simulink model "TraditionalStarterGenerator"  (R2024b)
settings: Solver=VariableStepAuto  StartTime=0.0  StopTime=20  MaxStep=1  RelTol=1e-3  EnableMultiTasking=on
undefined symbols (not defined in the file or in its folder): DiscIntNeverNeededParam
libraries: fl_lib x47, fl_ps_legacy_lib x26, ee_lib x25, nesl_utility x17, sdl_lib x1, SignalEditorBlockLib x1
(part 2 of 2)

== system TraditionalStarterGenerator/loads/Low Beam ==
  Fuse Right : ee_lib/Switches & Breakers/Fuse  prm=1  I_rated=15 A  melt_margin=1  T_fuse=0.5 s  I2t=1 s*A^2  I_vec=[1.9, 2.0, 2.5, 30.0] A  t_vec=[10000.0, 1.0, 0.3, 0.001] s  R_closed=0.01 Ohm  G_open=1e-8 1/Ohm  exposemeasurement=ee.enum.exposemeasurement.hidden
      settings: AttributesFormatString=%<I_rated> %<I_rated_unit>  InternalSimscapePortConfiguration="{\"Bottom\":[],\"Left\":[{\"id\":\"p\",\"label\":\"\",\"type\":\"foundation.electrical.electrical\"}],\"Right\":[{\"id\":\"n\",\"label\":\"\",\"type\":\"foundation.electrical.electrical\"}],\"Top\":[]}"
  Lamp : ee_lib/Passive/Incandescent Lamp  R_param=2  R0=0.15 Ohm  R1=1 Ohm  i0=5*25/12 A  i1=25/12 A  Vrated=12 V  alpha=0.004 1/K  tc=25 ms  initial_state=simscape.enum.onoff.off  t_fault=inf s
      settings: InternalSimscapePortConfiguration="{\"Bottom\":[],\"Left\":[{\"id\":\"p\",\"label\":\"+\",\"type\":\"foundation.electrical.electrical\"}],\"Right\":[{\"id\":\"n\",\"label\":\"-\",\"type\":\"foundation.electrical.electrical\"}],\"Top\":[]}"
  SPST Switch : ee_lib/Switches & Breakers/SPST Switch  R_closed=0.01 Ohm  G_open=1e-6 S  Threshold=0.5 V  Width=0 V  model_dynamics=0  t_on=1e-3 s  t_off=1e-3 s  initial_vT=0 V
      settings: InternalSimscapePortConfiguration="{\"Bottom\":[],\"Left\":[{\"id\":\"vT\",\"label\":\"vT\",\"type\":\"input\"},{\"id\":\"p\",\"label\":\"\",\"type\":\"foundation.electrical.electrical\"}],\"Right\":[{\"id\":\"n\",\"label\":\"\",\"type\":\"foundation.electrical.electrical\"}],\"Top\":[]}"
  Switch : PMIOPort  Side=Left
  - : PMIOPort  Port=2  Side=Right
  + : PMIOPort  Port=3  Side=Left
  connections:
  Fuse Right/RConn1 -- SPST Switch/LConn2
  SPST Switch/LConn1 -- Switch/RConn1
  SPST Switch/RConn1 -- Lamp/LConn1
  +/RConn1 -- Fuse Right/LConn1
  Lamp/RConn1 -- -/RConn1

== system TraditionalStarterGenerator/loads/Subsystem2 ==
  Simulink-PS Converter : nesl_utility/Simulink-PS Converter  PhysicalDomain=network_engine_domain  SubClassName=ps_input  LeftPortType=input  RightPortType=output  PseudoPeriodic=off  Frequencies=[]  NoiseDistribution=none  NoiseParameters=[]  Unit=1  AffineConversion=off  FilteringAndDerivatives=zero  SimscapeFilterOrder=1  InputFilterTimeConstant=0.001  UdotUserProvided=1
  ind_L : PMIOPort  Side=Right
  wires:
  [ind_L] -> Simulink-PS Converter/1
  connections:
  Simulink-PS Converter/RConn1 -- ind_L/RConn1

== system TraditionalStarterGenerator/loads/Subsystem3 ==
  Simulink-PS Converter : nesl_utility/Simulink-PS Converter  PhysicalDomain=network_engine_domain  SubClassName=ps_input  LeftPortType=input  RightPortType=output  PseudoPeriodic=off  Frequencies=[]  NoiseDistribution=none  NoiseParameters=[]  Unit=1  AffineConversion=off  FilteringAndDerivatives=zero  SimscapeFilterOrder=1  InputFilterTimeConstant=0.001  UdotUserProvided=1
  ind_R : PMIOPort  Side=Right
  wires:
  [ind_R] -> Simulink-PS Converter/1
  connections:
  Simulink-PS Converter/RConn1 -- ind_R/RConn1

== system TraditionalStarterGenerator/loads/Subsystem4 ==
  Simulink-PS Converter : nesl_utility/Simulink-PS Converter  PhysicalDomain=network_engine_domain  SubClassName=ps_input  LeftPortType=input  RightPortType=output  PseudoPeriodic=off  Frequencies=[]  NoiseDistribution=none  NoiseParameters=[]  Unit=1  AffineConversion=off  FilteringAndDerivatives=zero  SimscapeFilterOrder=1  InputFilterTimeConstant=0.001  UdotUserProvided=1
  lights : PMIOPort  Side=Right
  wires:
  [lights] -> Simulink-PS Converter/1
  connections:
  Simulink-PS Converter/RConn1 -- lights/RConn1

== system TraditionalStarterGenerator/loads/Subsystem5 ==
  Simulink-PS Converter : nesl_utility/Simulink-PS Converter  PhysicalDomain=network_engine_domain  SubClassName=ps_input  LeftPortType=input  RightPortType=output  PseudoPeriodic=off  Frequencies=[]  NoiseDistribution=none  NoiseParameters=[]  Unit=1  AffineConversion=off  FilteringAndDerivatives=zero  SimscapeFilterOrder=1  InputFilterTimeConstant=0.001  UdotUserProvided=1
  lights : PMIOPort  Side=Right
  wires:
  [lights] -> Simulink-PS Converter/1
  connections:
  Simulink-PS Converter/RConn1 -- lights/RConn1

== system TraditionalStarterGenerator/loads/Subsystem6 ==
  Simulink-PS Converter : nesl_utility/Simulink-PS Converter  PhysicalDomain=network_engine_domain  SubClassName=ps_input  LeftPortType=input  RightPortType=output  PseudoPeriodic=off  Frequencies=[]  NoiseDistribution=none  NoiseParameters=[]  Unit=1  AffineConversion=off  FilteringAndDerivatives=zero  SimscapeFilterOrder=1  InputFilterTimeConstant=0.001  UdotUserProvided=1
  brake : PMIOPort  Side=Right
  wires:
  [brake] -> Simulink-PS Converter/1
  connections:
  Simulink-PS Converter/RConn1 -- brake/RConn1

== system TraditionalStarterGenerator/loads/Subsystem7 ==
  Simulink-PS Converter : nesl_utility/Simulink-PS Converter  PhysicalDomain=network_engine_domain  SubClassName=ps_input  LeftPortType=input  RightPortType=output  PseudoPeriodic=off  Frequencies=[]  NoiseDistribution=none  NoiseParameters=[]  Unit=1  AffineConversion=off  FilteringAndDerivatives=zero  SimscapeFilterOrder=1  InputFilterTimeConstant=0.001  UdotUserProvided=1
  beam : PMIOPort  Side=Right
  wires:
  [beam] -> Simulink-PS Converter/1
  connections:
  Simulink-PS Converter/RConn1 -- beam/RConn1

== system TraditionalStarterGenerator/loads/Tail Light ==
  Fuse : ee_lib/Switches & Breakers/Fuse  prm=1  I_rated=5 A  melt_margin=1  T_fuse=0.5 s  I2t=1 s*A^2  I_vec=[1.9, 2.0, 2.5, 30.0] A  t_vec=[10000.0, 1.0, 0.3, 0.001] s  R_closed=0.01 Ohm  G_open=1e-8 1/Ohm  exposemeasurement=ee.enum.exposemeasurement.hidden
      settings: AttributesFormatString=%<I_rated> %<I_rated_unit>  InternalSimscapePortConfiguration="{\"Bottom\":[],\"Left\":[{\"id\":\"p\",\"label\":\"\",\"type\":\"foundation.electrical.electrical\"}],\"Right\":[{\"id\":\"n\",\"label\":\"\",\"type\":\"foundation.electrical.electrical\"}],\"Top\":[]}"
  Lamp : ee_lib/Passive/Incandescent Lamp  R_param=2  R0=0.15 Ohm  R1=1 Ohm  i0=5*5/12 A  i1=5/12 A  Vrated=12 V  alpha=0.004 1/K  tc=25 ms  initial_state=simscape.enum.onoff.off  t_fault=inf s
      settings: InternalSimscapePortConfiguration="{\"Bottom\":[],\"Left\":[{\"id\":\"p\",\"label\":\"+\",\"type\":\"foundation.electrical.electrical\"}],\"Right\":[{\"id\":\"n\",\"label\":\"-\",\"type\":\"foundation.electrical.electrical\"}],\"Top\":[]}"
  Switch SPST : ee_lib/Switches & Breakers/SPST Switch  R_closed=1 Ohm  G_open=1e-6 S  Threshold=0.5 V  Width=0 V  model_dynamics=0  t_on=0.001 s  t_off=0.001 s  initial_vT=0 V
      settings: InternalSimscapePortConfiguration="{\"Bottom\":[],\"Left\":[{\"id\":\"vT\",\"label\":\"vT\",\"type\":\"input\"},{\"id\":\"p\",\"label\":\"\",\"type\":\"foundation.electrical.electrical\"}],\"Right\":[{\"id\":\"n\",\"label\":\"\",\"type\":\"foundation.electrical.electrical\"}],\"Top\":[]}"
  Switch : PMIOPort  Side=Left
  + : PMIOPort  Port=2  Side=Left
  - : PMIOPort  Port=3  Side=Right
  connections:
  +/RConn1 -- Fuse/LConn1
  Lamp/RConn1 -- -/RConn1
  Switch/RConn1 -- Switch SPST/LConn1
  Fuse/RConn1 -- Switch SPST/LConn2
  Switch SPST/RConn1 -- Lamp/LConn1

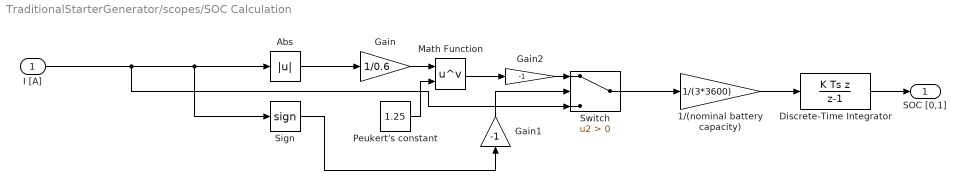
== system TraditionalStarterGenerator/scopes/SOC Calculation ==
  I [A] : Inport
  1/(nominal battery capacity) : Gain  Gain=1/(3*3600)
  Abs : Abs  SaturateOnIntegerOverflow=off
  Discrete-Time Integrator : DiscreteIntegrator  IntegratorMethod=Integration: Backward Euler  InitialCondition=0.5  SampleTime=0.0001  LimitOutput=on  UpperSaturationLimit=1  LowerSaturationLimit=0  ICPrevOutput=DiscIntNeverNeededParam  ICPrevScaledInput=DiscIntNeverNeededParam
  Gain : Gain  Gain=1/0.6
  Gain1 : Gain  Gain=-1
  Gain2 : Gain  Gain=-1
  Math Function : Math  Operator=pow
  Peukert's constant : Constant  Value=1.25  SampleTime=-1
  Sign : Signum
  Switch : Switch  Criteria=u2 > Threshold  SaturateOnIntegerOverflow=off  InputSameDT=off
  SOC [0,1] : Outport  VectorParamsAs1DForOutWhenUnconnected=off
  wires:
  Gain2/1 -> Switch/1
  Abs/1 -> Gain/1
  Discrete-Time Integrator/1 -> SOC [0,1]/1
  Sign/1 -> Gain1/1
  Math Function/1 -> Gain2/1
  I [A]/1 -> Sign/1, Abs/1, Switch/3
  Peukert's constant/1 -> Math Function/2
  Gain/1 -> Math Function/1
  Gain1/1 -> Switch/2
  Switch/1 -> 1/(nominal battery capacity)/1
  1/(nominal battery capacity)/1 -> Discrete-Time Integrator/1

== system TraditionalStarterGenerator/Alternator/Back EMF and Torque/Current Voltage Interface ==
  Controlled Voltage Source : fl_lib/Electrical/Electrical Sources/Controlled Voltage Source
  Current Sensor : fl_lib/Electrical/Electrical Sensors/Current Sensor
  v : PMIOPort  Side=Left
  i : PMIOPort  Port=2  Side=Right
  + : PMIOPort  Port=3  Side=Left
  - : PMIOPort  Port=4  Side=Right
  connections:
  Current Sensor/RConn1 -- i/RConn1
  Controlled Voltage Source/RConn1 -- v/RConn1
  Current Sensor/RConn2 -- Controlled Voltage Source/RConn2
  -/RConn1 -- Current Sensor/LConn1
  +/RConn1 -- Controlled Voltage Source/LConn1

== system TraditionalStarterGenerator/Alternator/Back EMF and Torque/Torque Motion Interface ==
  Motion Sensor : fl_lib/Mechanical/Mechanical Sensors/Ideal Rotational Motion Sensor  reference=foundation.enum.MeasurementReference.difference  acceleration_port=false  velocity_port=true  position_port=true  wrap_angle=simscape.enum.onoff.off  offset=0 rad
  Torque Source : fl_lib/Mechanical/Mechanical Sources/Ideal Torque Source
  C : PMIOPort  Side=Right
  R : PMIOPort  Port=2  Side=Left
  w : PMIOPort  Port=3  Side=Left
  trq : PMIOPort  Port=4  Side=Right
  connections:
  Motion Sensor/RConn2 -- w/RConn1
  trq/RConn1 -- Torque Source/RConn1
  Motion Sensor/LConn1 -- C/RConn1 -- Torque Source/RConn2
  Motion Sensor/RConn1 -- R/RConn1 -- Torque Source/LConn1

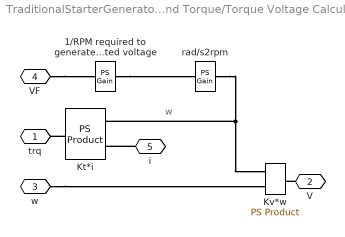
== system TraditionalStarterGenerator/Alternator/Back EMF and Torque/Torque Voltage Calculations ==
  note: w
  1/RPM required to generate rated voltage : fl_ps_legacy_lib/Legacy Physical Signals/Functions/PS Gain  gain=Kv
  Kt*i : fl_ps_legacy_lib/Legacy Physical Signals/Functions/PS Product
  Kv*w : fl_ps_legacy_lib/Legacy Physical Signals/Functions/PS Product
  rad/s2rpm : fl_ps_legacy_lib/Legacy Physical Signals/Functions/PS Gain  gain=60/(2*pi)
  trq : PMIOPort  Side=Left
  V : PMIOPort  Port=2  Side=Right
  w : PMIOPort  Port=3  Side=Left
  VF : PMIOPort  Port=4  Side=Left
  i : PMIOPort  Port=5  Side=Right
  connections:
  rad/s2rpm/RConn1 -- Kv*w/LConn1 -- Kt*i/LConn2
  1/RPM required to generate rated voltage/RConn1 -- rad/s2rpm/LConn1
  i/RConn1 -- Kt*i/LConn1
  V/RConn1 -- Kv*w/RConn1
  VF/RConn1 -- 1/RPM required to generate rated voltage/LConn1
  w/RConn1 -- Kv*w/LConn2
  Kt*i/RConn1 -- trq/RConn1

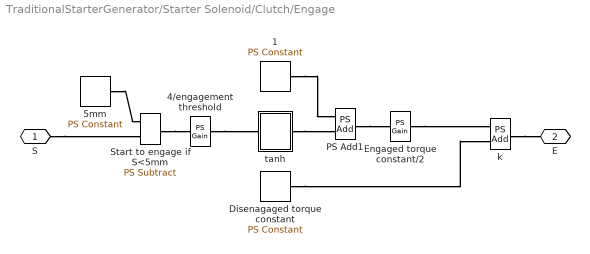
== system TraditionalStarterGenerator/Starter Solenoid/Clutch/Engage ==
  1 : fl_lib/Physical Signals/Sources/PS Constant  constant=1
  4/engagement threshold : fl_ps_legacy_lib/Legacy Physical Signals/Functions/PS Gain  gain=4/1e-3
  5mm : fl_lib/Physical Signals/Sources/PS Constant  constant=5e-3
  Disenagaged torque constant : fl_lib/Physical Signals/Sources/PS Constant  constant=1e-8
  Engaged torque constant/2 : fl_ps_legacy_lib/Legacy Physical Signals/Functions/PS Gain  gain=500/2
  PS Add1 : fl_ps_legacy_lib/Legacy Physical Signals/Functions/PS Add
      settings: InternalSimscapePortConfiguration="{\"Bottom\":[],\"Left\":[{\"id\":\"I1\",\"label\":\"\",\"type\":\"input\"},{\"id\":\"I2\",\"label\":\"\",\"type\":\"input\"}],\"Right\":[{\"id\":\"O\",\"label\":\"\",\"type\":\"output\"}],\"Top\":[]}"
  Start to engage if S<5mm : fl_ps_legacy_lib/Legacy Physical Signals/Functions/PS Subtract
  k : fl_ps_legacy_lib/Legacy Physical Signals/Functions/PS Add
      settings: InternalSimscapePortConfiguration="{\"Bottom\":[],\"Left\":[{\"id\":\"I1\",\"label\":\"\",\"type\":\"input\"},{\"id\":\"I2\",\"label\":\"\",\"type\":\"input\"}],\"Right\":[{\"id\":\"O\",\"label\":\"\",\"type\":\"output\"}],\"Top\":[]}"
  tanh : Subsystem
  S : PMIOPort  Side=Left
  E : PMIOPort  Port=2  Side=Right
  connections:
  S/RConn1 -- Start to engage if S<5mm/LConn2
  5mm/RConn1 -- Start to engage if S<5mm/LConn1
  1/RConn1 -- PS Add1/LConn1
  Disenagaged torque constant/RConn1 -- k/LConn2
  PS Add1/RConn1 -- Engaged torque constant/2/LConn1
  Engaged torque constant/2/RConn1 -- k/LConn1
  4/engagement threshold/RConn1 -- tanh/LConn1
  tanh/RConn1 -- PS Add1/LConn2
  Start to engage if S<5mm/RConn1 -- 4/engagement threshold/LConn1
  k/RConn1 -- E/RConn1

== system TraditionalStarterGenerator/loads/Indicators/Blinker ==
  Pulse Generator : DiscretePulseGenerator  PulseType=Time based  Period=1.5  PulseWidth=50
  Rate Transition : RateTransition
  SPST Switch1 : ee_lib/Switches & Breakers/SPST Switch  R_closed=1 Ohm  G_open=1e-6 S  Threshold=0.5 V  Width=0 V  model_dynamics=0  t_on=0.001 s  t_off=0.001 s  initial_vT=0 V
      settings: InternalSimscapePortConfiguration="{\"Bottom\":[],\"Left\":[{\"id\":\"vT\",\"label\":\"vT\",\"type\":\"input\"},{\"id\":\"p\",\"label\":\"\",\"type\":\"foundation.electrical.electrical\"}],\"Right\":[{\"id\":\"n\",\"label\":\"\",\"type\":\"foundation.electrical.electrical\"}],\"Top\":[]}"
  Simulink-PS Converter : nesl_utility/Simulink-PS Converter  PhysicalDomain=network_engine_domain  SubClassName=ps_input  LeftPortType=input  RightPortType=output  PseudoPeriodic=off  Frequencies=[]  NoiseDistribution=none  NoiseParameters=[]  Unit=1  AffineConversion=off  FilteringAndDerivatives=zero  SimscapeFilterOrder=1  InputFilterTimeConstant=0.001  UdotUserProvided=1
  + : PMIOPort  Side=Left
  - : PMIOPort  Port=2  Side=Right
  wires:
  Pulse Generator/1 -> Rate Transition/1
  Rate Transition/1 -> Simulink-PS Converter/1
  connections:
  +/RConn1 -- SPST Switch1/LConn2
  SPST Switch1/RConn1 -- -/RConn1
  Simulink-PS Converter/RConn1 -- SPST Switch1/LConn1

== system TraditionalStarterGenerator/Starter Solenoid/Clutch/Engage/tanh ==
  -2u : fl_ps_legacy_lib/Legacy Physical Signals/Functions/PS Gain  gain=-2
  1 : fl_lib/Physical Signals/Sources/PS Constant  constant=1
  PS Add : fl_ps_legacy_lib/Legacy Physical Signals/Functions/PS Add
      settings: InternalSimscapePortConfiguration="{\"Bottom\":[],\"Left\":[{\"id\":\"I1\",\"label\":\"\",\"type\":\"input\"},{\"id\":\"I2\",\"label\":\"\",\"type\":\"input\"}],\"Right\":[{\"id\":\"O\",\"label\":\"\",\"type\":\"output\"}],\"Top\":[]}"
  PS Divide : fl_ps_legacy_lib/Legacy Physical Signals/Functions/PS Divide
      settings: InternalSimscapePortConfiguration="{\"Bottom\":[],\"Left\":[{\"id\":\"I1\",\"label\":\"\",\"type\":\"input\"},{\"id\":\"I2\",\"label\":\"\",\"type\":\"input\"}],\"Right\":[{\"id\":\"O\",\"label\":\"\",\"type\":\"output\"}],\"Top\":[]}"
  PS Subtract : fl_ps_legacy_lib/Legacy Physical Signals/Functions/PS Subtract
  exp(-2*u) : fl_ps_legacy_lib/Legacy Physical Signals/Functions/PS Math Function  fcn_choice=3
      settings: InternalSimscapePortConfiguration="{\"Bottom\":[],\"Left\":[{\"id\":\"I\",\"label\":\"\",\"type\":\"input\"}],\"Right\":[{\"id\":\"O\",\"label\":\"\",\"type\":\"output\"}],\"Top\":[]}"
  u : PMIOPort  Side=Left
  y : PMIOPort  Port=2  Side=Right
  connections:
  -2u/RConn1 -- exp(-2*u)/LConn1
  u/RConn1 -- -2u/LConn1
  exp(-2*u)/RConn1 -- PS Add/LConn2 -- PS Subtract/LConn2
  1/RConn1 -- PS Subtract/LConn1 -- PS Add/LConn1
  PS Subtract/RConn1 -- PS Divide/LConn1
  PS Add/RConn1 -- PS Divide/LConn2
  PS Divide/RConn1 -- y/RConn1
